simulink model "direct_form2"  (R2014b)
settings: Solver=ode45  StartTime=0.0  StopTime=10.0  RelTol=1e-3
settings Model: Creator=ravoson  LastModifiedBy=ravoson

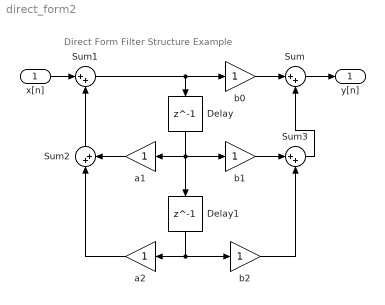
== system direct_form2 ==
  note: Direct Form Filter Structure Example
  x[n] : Inport
  Delay : Delay  DelayLength=1  InitialCondition=0
  Delay1 : Delay  DelayLength=1  InitialCondition=0
  Sum{,1..3} (4 alike) : Sum  Inputs=|++
  a1 : Gain
  a2 : Gain
  b0 : Gain
  b1 : Gain
  b2 : Gain
  y[n] : Outport
  wires:
  x[n]/1 -> Sum1/1
  Sum1/1 -> Delay/1, b0/1
  b0/1 -> Sum/1
  Sum/1 -> y[n]/1
  Sum2/1 -> Sum1/2
  a1/1 -> Sum2/2
  Delay/1 -> Delay1/1, b1/1, a1/1
  Delay1/1 -> b2/1, a2/1
  a2/1 -> Sum2/1
  Sum3/1 -> Sum/2
  b1/1 -> Sum3/1
  b2/1 -> Sum3/2
